simulink model "sampleModel309"  (R2021b)
settings: Solver=VariableStepAuto  StartTime=0.0  StopTime=10.0  RelTol=1e-3
undefined symbols (not defined in the file or in its folder): DiscIntNeverNeededParam
libraries: simulink x6, slpidlib x1
settings Model: Creator=user  LastModifiedBy=user

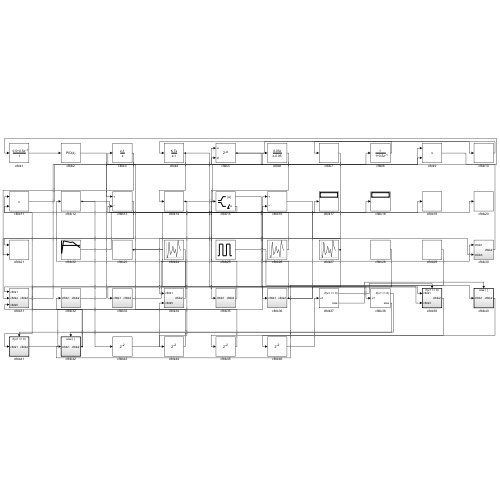
[thumbnail: Simulink's stored preview of the top-level diagram]
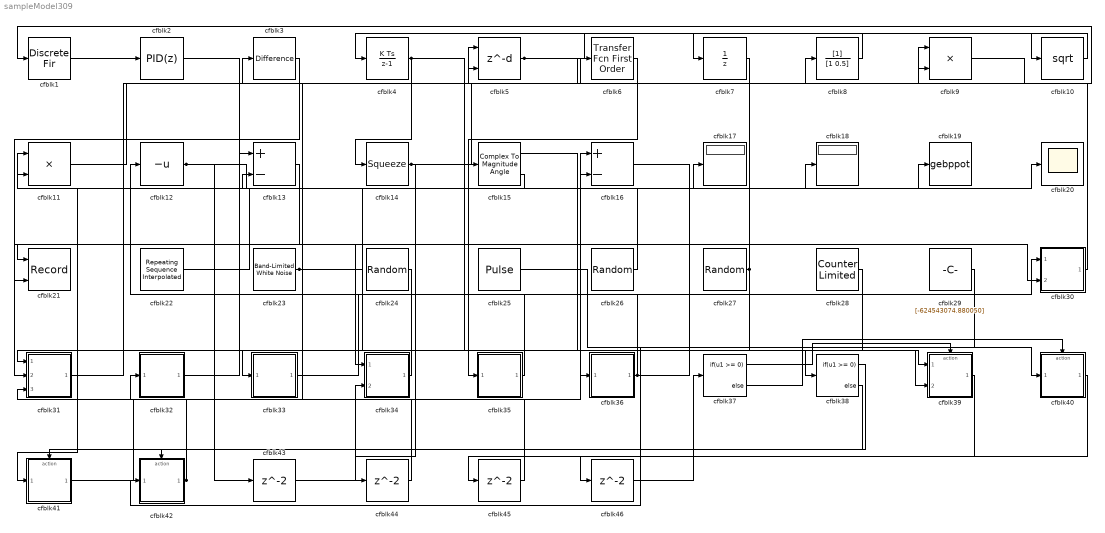
== system sampleModel309 ==
  cfblk1 : DiscreteFir  SampleTime=1
  cfblk10 : Sqrt  SaturateOnIntegerOverflow=on
  cfblk11 : Product  Inputs=**
  cfblk12 : UnaryMinus
  cfblk13 : Sum  Inputs=+-
  cfblk14 : Squeeze
  cfblk15 : ComplexToMagnitudeAngle
  cfblk16 : Sum  Inputs=+-
  cfblk17 : Display
  cfblk18 : Display
  cfblk19 : ToWorkspace  VariableName=gebppot  SaveFormat=Timeseries  SampleTime=-1
  cfblk2 : slpidlib/PID Controller  Controller=PID  Form=Parallel  TimeDomain=Discrete-time  UseExternalTs=off  SampleTime=1  IntegratorMethod=Forward Euler  FilterMethod=Forward Euler  ControllerParametersSource=internal  P=1  I=1  D=0  UseFilter=on  N=100  TunerSelectOption=Transfer Function Based (PID Tuner App)  InitialConditionSource=internal  InitialConditionForIntegrator=0  InitialConditionForFilter=0  DifferentiatorICPrevScaledInput=0  ExternalReset=none  TrackingMode=off  Kt=1  LimitOutput=off  SatLimitsSource=internal  UpperSaturationLimit=inf  LowerSaturationLimit=-inf  LinearizeAsGain=off  AntiWindupMode=none  Kb=1  POutMin=[]  POutMax=[]  IOutMin=[]  IOutMax=[]  DOutMin=[]  DOutMax=[]  NOutMin=[]  NOutMax=[]  SumOutMin=[]  SumOutMax=[]  SaturationOutMin=[]  SaturationOutMax=[]  PParamMin=[]  PParamMax=[]  IParamMin=[]  IParamMax=[]  DParamMin=[]  DParamMax=[]  NParamMin=[]  NParamMax=[]  KbParamMin=[]  KbParamMax=[]  KtParamMin=[]  KtParamMax=[]  KbOutMin=[]  KbOutMax=[]  KtOutMin=[]  KtOutMax=[]  IntegratorOutMin=[]  IntegratorOutMax=[]  FilterOutMin=[]  FilterOutMax=[]  SumI1OutMin=[]  SumI1OutMax=[]  SumI2OutMin=[]  SumI2OutMax=[]  SumI3OutMin=[]  SumI3OutMax=[]  SumI4OutMin=[]  SumI4OutMax=[]  SumDOutMin=[]  SumDOutMax=[]  DifferentiatorOutMin=[]  DifferentiatorOutMax=[]  FilterDiffOutCoefMin=[]  FilterDiffOutCoefMax=[]  ReciprocalOutMin=[]  ReciprocalOutMax=[]  SumDenOutMin=[]  SumDenOutMax=[]  SumNumOutMin=[]  SumNumOutMax=[]  DivideOutMin=[]  DivideOutMax=[]  UdiffTsProdOutMin=[]  UdiffTsProdOutMax=[]  NTsProdOutMin=[]  NTsProdOutMax=[]  UintegralTsProdOutMin=[]  UintegralTsProdOutMax=[]  UngainTsProdOutMin=[]  UngainTsProdOutMax=[]  IntegratorContinuousStateAttributes=''  IntegratorStateMustResolveToSignalObject=off  IntegratorRTWStateStorageClass=Auto  FilterContinuousStateAttributes=''  FilterStateMustResolveToSignalObject=off  FilterRTWStateStorageClass=Auto  ParallelPVariant=InternalParameters  IdealPVariant=Disabled  IVariant=InternalParameters  DVariant=InternalParameters  IntegratorVariant=Discrete  SatVariant=Disabled  AWVariant=Passthrough  PCopyVariant=Disabled  TRVariant=Disabled  FdbkBlocksVariant=Forward  IdealPFdbkVariant=Disabled  SatFdbkVariant=Disabled  DerivativeFilterVariant=ForwardEulerFilter  NVariant=InternalParameters  NCopyVariant=Disabled  FilterICVariant=InternalICsFilter  IntegratorICVariant=InternalICs  ExternalResetVariant=Disabled  TRSumVariant=Passthrough  SumFdbkVariant=Disabled  SumVariant=Sum_PID  TsampFilterVariant=InternalTs  TsampNgainVariant=Passthrough  TsampIntegralVariant=Passthrough  ExternalSaturationOutDataTypeStr=Inherit: Same as second input
  cfblk20 : Scope
  cfblk21 : Record  FileSettingsInternal="{\"entries\":[{\"content\":{\"excelSettings\":{\"content\":{},\"type\":\"Streamout.ExcelSettings\"}},\"type\":\"Streamout.FileSettingStorage\",\"uuid\":\"e8b4a27f-2ffb-462a-82d9-dfe7f21218f6\"}],\"packageUris\":[\"http://schema.mathworks.com/mf0/streamout_blocks/R2020a\"],\"version\":\"1.0\"}"  Layout=[1 1]  SignalsInternal="{\"entries\":[{\"content\":{\"signals\":[{\"content\":{\"blockPath\":[\"sampleModel309/cfblk21\"],\"channel\":[],\"dimensions\":[1],\"domain\":\"sampleModel309/cfblk21\",\"lineColor\":\"#a2142f\",\"plots\":[1],\"port\":1,\"sid\":[\"\"],\"signalID\":13115,\"signalName\":\"cfblk27\"},\"type\":\"RecordBlkView.Signal\",\"uuid\":\"bc8db662-9bde-4065-99a0-26c4efb5457f\"},{\"content\":{\"blockPath\":[\"sampleModel309/cfblk21\"],\"channel\":[],\"dimensions\":[1],\"domain\":\"sampleModel309/cfblk21\",\"lineColor\":\"#139fff\",\"plots\":[1],\"port\":2,\"sid\":[\"\"],\"signalID\":13119,\"signalName\":\"cfblk13\"},\"type\":\"RecordBlkView.Signal\",\"uuid\":\"61146a21-7cf5-44f0-a458-61e732db696e\"}]},\"type\":\"RecordBlkView.InputSignals\",\"uuid\":\"9cc0d5da-ed63-415b-bfb5-34102d37701a\"}],\"packageUris\":[\"http://schema.mathworks.com/mf0/streamout_blocks/R2020a\"],\"version\":\"1.0\"}"  VisualizationBindings="{\"xyplotplugin\":{\"info\":[{\"series\":[{\"bindingParametersList\":[{\"parameter\":\"X-Axis\",\"signalID\":13115,\"signalName\":\"cfblk27\"},{\"parameter\":\"Y-Axis\",\"signalID\":13119,\"signalName\":\"cfblk13\"}],\"seriesID\":30490}],\"subplotID\":1}]}}"  CompatibilityTag=XY
  cfblk22 : simulink/Sources/Repeating Sequence Interpolated  OutValues=[-833607402.613657, 483514591.781908, 308594911.286002, 385882726.624820, -231198009.761560]  TimeValues=[0 0.1 0.5 0.6 1].'  LookUpMeth=Use Input Below  tsamp=0.01  OutMin=[]  OutMax=[]  OutDataTypeStr=double  OutputDataTypeScalingMode=double  OutDataType=fixdt(0,8)  OutScaling=2^-10
  cfblk23 : simulink/Sources/Band-Limited White Noise  Cov=[110730013.501640]  Ts=0.1  seed=[9650357808.000000]
  cfblk24 : UniformRandomNumber  Minimum=[-9278582345.539703]  Maximum=[7160088709.474762]  Seed=[44375776.000000]  SampleTime=0.1
  cfblk25 : DiscretePulseGenerator  PulseType=Time based  Amplitude=[-576541843.015773]  Period=[75631927.515971]  PulseWidth=5  PhaseDelay=[6.000000]
  cfblk26 : UniformRandomNumber  Minimum=[-2680244145.848851]  Maximum=[2925774436.473303]  Seed=[59871340.000000]  SampleTime=0.1
  cfblk27 : UniformRandomNumber  Minimum=[-5734100249.088449]  Maximum=[31166541.110866]  Seed=[53513765.000000]  SampleTime=0.1
  cfblk28 : simulink/Sources/Counter Limited  uplimit=[728.000000]  tsamp=-1
  cfblk29 : Constant  Value=[-624543074.880050]  SampleTime=1
  cfblk3 : simulink/Discrete/Difference  ICPrevInput=0.0  OutMin=[]  OutMax=[]  OutDataTypeStr=Inherit: Inherit via back propagation  OutDataType=fixdt(1, 16)  OutScaling=2^-10  DoSatur=off
  cfblk30 : Subsystem
  cfblk31 : Subsystem
  cfblk32 : Subsystem
  cfblk33 : Subsystem
  cfblk34 : Subsystem
  cfblk35 : Subsystem
  cfblk36 : Subsystem
  cfblk37 : If  IfExpression=u1 >= 0  SampleTime=1
  cfblk38 : If  IfExpression=u1 >= 0  SampleTime=1
  cfblk39 : Subsystem  TreatAsAtomicUnit=on
  cfblk4 : DiscreteIntegrator  ICPrevOutput=DiscIntNeverNeededParam  ICPrevScaledInput=DiscIntNeverNeededParam
  cfblk40 : Subsystem  TreatAsAtomicUnit=on
  cfblk41 : Subsystem  TreatAsAtomicUnit=on
  cfblk42 : Subsystem  TreatAsAtomicUnit=on
  cfblk{43..46} (4 alike) : Delay  SampleTime=1
  cfblk5 : Delay  DelayLengthSource=Input port  SampleTime=1
      settings: InputPortMap=u0,p1
  cfblk6 : simulink/Discrete/Transfer Fcn First Order  PoleZ=0.95  ICPrevOutput=0.0  DoSatur=off
  cfblk7 : UnitDelay  HasFrameUpgradeWarning=on
  cfblk8 : DiscreteFilter  SampleTime=1
  cfblk9 : Product  Inputs=**
  wires:
  cfblk23/1 -> cfblk18/1, cfblk36/1(cfblk1)
  cfblk34/1(cfblk2) -> cfblk12/1
  cfblk14/1 -> cfblk8/1, cfblk44/1
  cfblk5/1 -> cfblk10/1, cfblk9/2
  cfblk42/1(cfblk2) -> cfblk32/1(cfblk1), cfblk11/2
  cfblk31/1(cfblk2) -> cfblk5/1
  cfblk41/1(cfblk2) -> cfblk16/1
  cfblk29/1 -> cfblk42/1(cfblk1)
  cfblk25/1 -> cfblk40/1(cfblk1)
  cfblk9/1 -> cfblk1/1
  cfblk28/1 -> cfblk31/1(cfblk1)
  cfblk6/1 -> cfblk35/1(cfblk1)
  cfblk4/1 -> cfblk14/1, cfblk39/2(cfblk3)
  cfblk33/1(cfblk2) -> cfblk30/1(cfblk1)
  cfblk2/1 -> cfblk13/1
  cfblk1/1 -> cfblk2/1
  cfblk12/1 -> cfblk17/1, cfblk43/1
  cfblk16/1 -> cfblk30/2(cfblk3)
  cfblk30/1(cfblk2) -> cfblk5/2
  cfblk36/1(cfblk2) -> cfblk16/2, cfblk20/1, cfblk38/1
  cfblk35/1(cfblk2) -> cfblk15/1
  cfblk3/1 -> cfblk31/2(cfblk4)
  cfblk27/1 -> cfblk21/1, cfblk41/1(cfblk1)
  cfblk8/1 -> cfblk7/1
  cfblk24/1 -> cfblk33/1(cfblk1)
  cfblk15/1 -> cfblk39/1(cfblk1)
  cfblk10/1 -> cfblk4/1
  cfblk11/1 -> cfblk6/1
  cfblk32/1(cfblk2) -> cfblk9/1
  cfblk13/1 -> cfblk21/2
  cfblk22/1 -> cfblk19/1
  cfblk26/1 -> cfblk11/1
  cfblk7/1 -> cfblk34/1(cfblk1)
  cfblk15/2 -> cfblk13/2
  cfblk37/1 -> cfblk39/Action
  cfblk37/2 -> cfblk40/Action
  cfblk38/1 -> cfblk41/Action
  cfblk38/2 -> cfblk42/Action
  cfblk43/1 -> cfblk34/2(cfblk5)
  cfblk44/1 -> cfblk31/3(cfblk5)
  cfblk39/1(cfblk2) -> cfblk45/1
  cfblk45/1 -> cfblk3/1
  cfblk40/1(cfblk2) -> cfblk46/1
  cfblk46/1 -> cfblk37/1

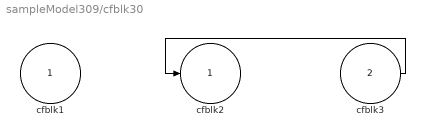
== system sampleModel309/cfblk30 ==
  cfblk1 : Inport
  cfblk3 : Inport  Port=2
  cfblk2 : Outport
  wires:
  cfblk3/1 -> cfblk2/1

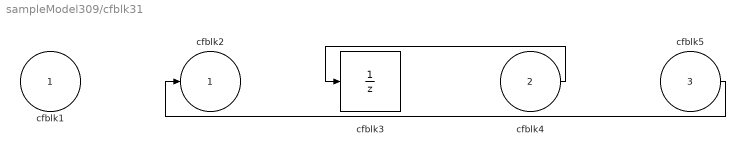
== system sampleModel309/cfblk31 ==
  cfblk1 : Inport
  cfblk4 : Inport  Port=2
  cfblk5 : Inport  Port=3
  cfblk3 : UnitDelay  HasFrameUpgradeWarning=on
  cfblk2 : Outport
  wires:
  cfblk4/1 -> cfblk3/1
  cfblk5/1 -> cfblk2/1

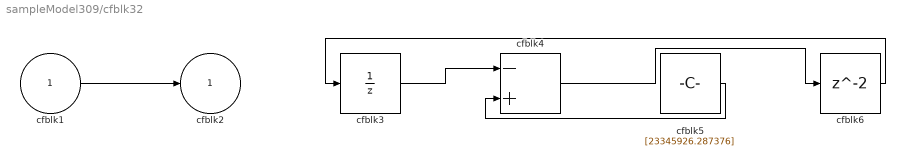
== system sampleModel309/cfblk32 ==
  cfblk1 : Inport
  cfblk3 : UnitDelay  HasFrameUpgradeWarning=on
  cfblk4 : Sum  Inputs=-+
  cfblk5 : Constant  Value=[23345926.287376]  SampleTime=1
  cfblk6 : Delay  SampleTime=1
  cfblk2 : Outport
  wires:
  cfblk3/1 -> cfblk4/1
  cfblk1/1 -> cfblk2/1
  cfblk5/1 -> cfblk4/2
  cfblk4/1 -> cfblk6/1
  cfblk6/1 -> cfblk3/1

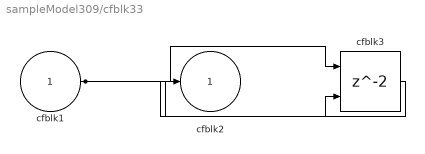
== system sampleModel309/cfblk33 ==
  cfblk1 : Inport
  cfblk3 : Delay  ShowEnablePort=on  SampleTime=1
      settings: InputPortMap=u0,e6
  cfblk2 : Outport
  wires:
  cfblk1/1 -> cfblk3/1, cfblk3/2
  cfblk3/1 -> cfblk2/1

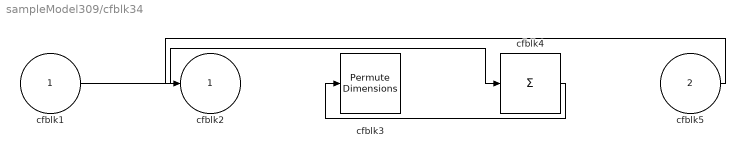
== system sampleModel309/cfblk34 ==
  cfblk1 : Inport
  cfblk5 : Inport  Port=2
  cfblk3 : PermuteDimensions
  cfblk4 : Sum  Inputs=+
  cfblk2 : Outport
  wires:
  cfblk1/1 -> cfblk4/1
  cfblk4/1 -> cfblk3/1
  cfblk5/1 -> cfblk2/1

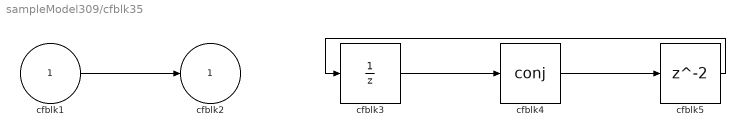
== system sampleModel309/cfblk35 ==
  cfblk1 : Inport
  cfblk3 : UnitDelay  HasFrameUpgradeWarning=on
  cfblk4 : Math  Operator=conj  SaturateOnIntegerOverflow=on
  cfblk5 : Delay  SampleTime=1
  cfblk2 : Outport
  wires:
  cfblk1/1 -> cfblk2/1
  cfblk3/1 -> cfblk4/1
  cfblk4/1 -> cfblk5/1
  cfblk5/1 -> cfblk3/1

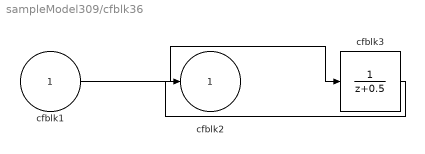
== system sampleModel309/cfblk36 ==
  cfblk1 : Inport
  cfblk3 : DiscreteTransferFcn  SampleTime=1
  cfblk2 : Outport
  wires:
  cfblk1/1 -> cfblk3/1
  cfblk3/1 -> cfblk2/1

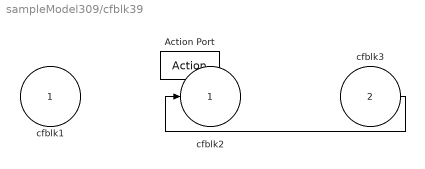
== system sampleModel309/cfblk39 ==
  cfblk1 : Inport
  cfblk3 : Inport  Port=2
  Action Port : ActionPort  ActionPortLabel=if(u1 >= 0)
  cfblk2 : Outport
  wires:
  cfblk3/1 -> cfblk2/1

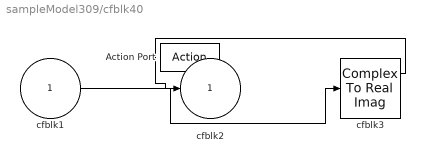
== system sampleModel309/cfblk40 ==
  cfblk1 : Inport
  Action Port : ActionPort  ActionPortLabel=else
  cfblk3 : ComplexToRealImag
  cfblk2 : Outport
  wires:
  cfblk1/1 -> cfblk3/1
  cfblk3/1 -> cfblk2/1

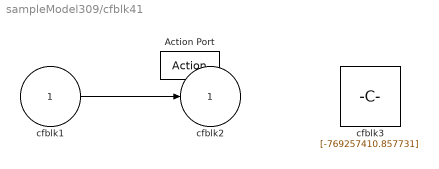
== system sampleModel309/cfblk41 ==
  cfblk1 : Inport
  Action Port : ActionPort  ActionPortLabel=if(u1 >= 0)
  cfblk3 : Constant  Value=[-769257410.857731]  SampleTime=1
  cfblk2 : Outport
  wires:
  cfblk1/1 -> cfblk2/1

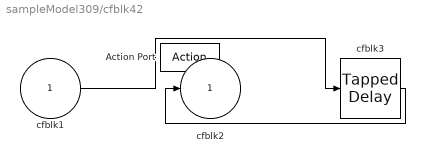
== system sampleModel309/cfblk42 ==
  cfblk1 : Inport
  Action Port : ActionPort  ActionPortLabel=else
  cfblk3 : simulink/Discrete/Tapped Delay  vinit=0.0  samptime=-1  NumDelays=1  DelayOrder=Oldest  includeCurrent=off
  cfblk2 : Outport
  wires:
  cfblk3/1 -> cfblk2/1
  cfblk1/1 -> cfblk3/1
